simulink model "ej_07_simulink"  (R2022b)
settings: Solver=VariableStepAuto  StartTime=0.0  StopTime=2.5  RelTol=1e-3
values from neighbouring files (symbols this model uses):
  X0 = [-1 1]    [ej_07.m]    (also in ej_08.m = [1 0 0]; ej_09.m = 0)
libraries: MainLibrary x1
settings Model: Creator=cotti  LastModifiedBy=cotti

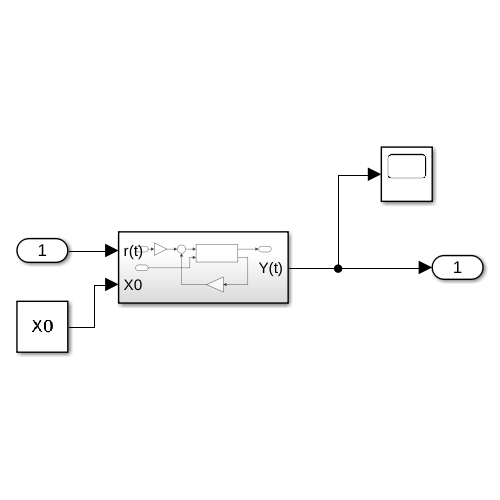
[thumbnail: Simulink's stored preview of the top-level diagram]
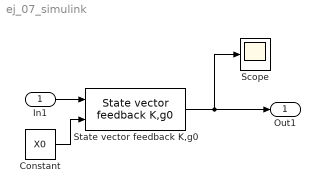
== system ej_07_simulink ==
  In1 : Inport
  Constant : Constant  Value=X0
  Scope : Scope
  State vector feedback K,g0 : MainLibrary/State vector feedback K,g0  SystemSampleTime=-1  VariantActivationTime=update diagram  Latency=0  AutoFrameSizeCalculation=off
  Out1 : Outport
  wires:
  In1/1 -> State vector feedback K,g0/1
  State vector feedback K,g0/1 -> Scope/1, Out1/1
  Constant/1 -> State vector feedback K,g0/2
